simulink model "BFSK"  (R2021a)
settings: Solver=VariableStepAuto  StartTime=0.0  StopTime=10.0  RelTol=1e-3
libraries: commdigbbndfm2 x4, commchan3 x2, commsink2 x2, commrandsrc3 x2, dspsigops x1, dspquant2 x1
settings Model: Creator=Bharat Gunhalkar  LastModifiedBy=Bharat Gunhalkar

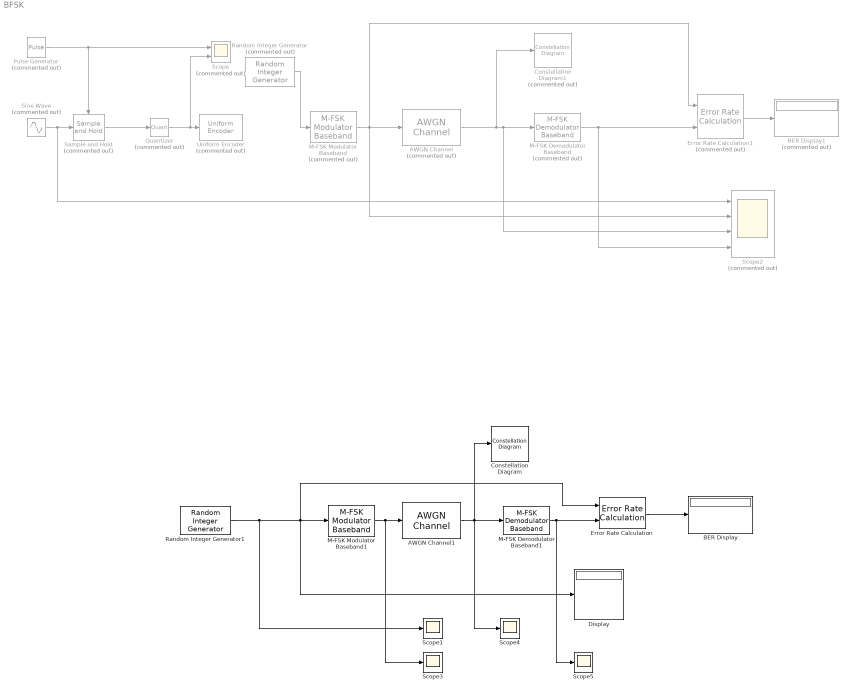
== system BFSK ==
  AWGN Channel : commchan3/AWGN Channel  Commented=on  InputProcessing=Columns as channels (frame based)  seed=67  noiseMode="Signal to noise ratio  (Eb/No)"  EbNodB=10  EsNodB=10  SNRdB=10  bitsPerSym=1  Ps=1  Tsym=1  variance=1
  AWGN Channel1 : commchan3/AWGN Channel  InputProcessing=Columns as channels (frame based)  seed=67  noiseMode="Signal to noise ratio  (Eb/No)"  EbNodB=1  EsNodB=10  SNRdB=10  bitsPerSym=1  Ps=1  Tsym=1  variance=1
  BER Display : Display
  BER Display1 : Display  Commented=on
  Constellation Diagram : ConstellationDiagram
  Constellation Diagram1 : ConstellationDiagram  Commented=on
  Display : Display
  Error Rate Calculation : commsink2/Error Rate Calculation  N=0  st_delay=0  cp_mode=Entire frame  subframe=[]  PMode=Port  WsName=ErrorVec  RsMode2=off  stop=off  numErr=100  maxBits=1e6
  Error Rate Calculation1 : commsink2/Error Rate Calculation  Commented=on  N=0  st_delay=0  cp_mode=Entire frame  subframe=[]  PMode=Port  WsName=ErrorVec  RsMode2=off  stop=off  numErr=100  maxBits=1e6
  M-FSK Demodulator Baseband : commdigbbndfm2/M-FSK Demodulator Baseband  Commented=on  M=8  OutType=Integer  Dec=Gray  freqSep=6  numSamp=17  RateOptions=Enforce single-rate processing  outDataType=double
      settings: SourceProductBaseCode=CM
  M-FSK Demodulator Baseband1 : commdigbbndfm2/M-FSK Demodulator Baseband  M=8  OutType=Integer  Dec=Gray  freqSep=6  numSamp=17  RateOptions=Enforce single-rate processing  outDataType=double
      settings: SourceProductBaseCode=CM
  M-FSK Modulator Baseband : commdigbbndfm2/M-FSK Modulator Baseband  Commented=on  M=8  InType=Integer  Enc=Gray  freqSep=6  phaseType=Continuous  numSamp=17  RateOptions=Enforce single-rate processing  outDataType=double
  M-FSK Modulator Baseband1 : commdigbbndfm2/M-FSK Modulator Baseband  M=8  InType=Integer  Enc=Gray  freqSep=6  phaseType=Continuous  numSamp=17  RateOptions=Enforce single-rate processing  outDataType=double
  Pulse Generator : DiscretePulseGenerator  Commented=on  Period=1000  PulseWidth=5
  Quantizer : Quantizer  Commented=on  QuantizationInterval=.125  LinearizeAsGain=off
  Random Integer Generator : commrandsrc3/Random Integer Generator  Commented=on  SetSize=8  SeedSource=Auto  Seed=0  SampleTime=1  SamplesPerFrame=100  OutputDataType=double  SimulateUsing=Interpreted execution
  Random Integer Generator1 : commrandsrc3/Random Integer Generator  SetSize=8  SeedSource=Auto  Seed=0  SampleTime=1  SamplesPerFrame=100  OutputDataType=double  SimulateUsing=Interpreted execution
  Sample and Hold : dspsigops/Sample and Hold  Commented=on  trig=Rising edge  initCond=0  latchinput=off
  Scope : Scope  Commented=on  NumInputPorts=2
  Scope{1,3..5} (4 alike) : Scope
  Scope2 : Scope  Commented=on  NumInputPorts=4
  Sine Wave : Sin  Commented=on  Amplitude=10  SampleTime=0
  Uniform Encoder : dspquant2/Uniform Encoder  Commented=on  peak=1  bits=8  otype=Unsigned integer
  wires:
  M-FSK Demodulator Baseband/1 -> Error Rate Calculation1/2, Scope2/4
  Quantizer/1 -> Scope/2, Uniform Encoder/1
  Pulse Generator/1 -> Sample and Hold/Trigger, Scope/1
  Sample and Hold/1 -> Quantizer/1
  Sine Wave/1 -> Scope2/1, Sample and Hold/1
  M-FSK Modulator Baseband/1 -> AWGN Channel/1, Scope2/2, Error Rate Calculation1/1
  Error Rate Calculation1/1 -> BER Display1/1
  Random Integer Generator/1 -> M-FSK Modulator Baseband/1
  AWGN Channel/1 -> Scope2/3, M-FSK Demodulator Baseband/1, Constellation Diagram1/1
  M-FSK Modulator Baseband1/1 -> Scope3/1, AWGN Channel1/1
  Error Rate Calculation/1 -> BER Display/1
  M-FSK Demodulator Baseband1/1 -> Scope5/1, Error Rate Calculation/2
  AWGN Channel1/1 -> Scope4/1, M-FSK Demodulator Baseband1/1, Constellation Diagram/1
  Random Integer Generator1/1 -> Scope1/1, Display/1, Error Rate Calculation/1, M-FSK Modulator Baseband1/1
